simulink model "signal_proc"  (R2017a)
settings: Solver=VariableStepAuto  StartTime=0.0  StopTime=50  RelTol=1e-3  EnableMultiTasking=on
values from neighbouring files (symbols this model uses):
  Ts = 1/ Fs    (= 0.008)    [example_1.m]    (also in my_filter.m = 1/Fs)
libraries: dspsrcs4 x1
settings Model: Creator=haroldfmurcia  LastModifiedBy=root
settings OptimizationCC: LifeSpan=inf
settings DebuggingCC: SFUnexpectedBacktrackingDiag=warning  SFNoUnconditionalDefaultTransitionDiag=warning  SFExecutionAtInitializationDiag=none
settings GRTTargetCC: TargetLangStandard=C89/C90 (ANSI)  GeneratePreprocessorConditionals=Disable all
settings ConfigComp: CovMetricSettings=dw  CovHtmlReporting=on  CovSaveCumulativeToWorkspaceVar=on  CovSaveSingleToWorkspaceVar=on  CovExternalEMLEnable=off

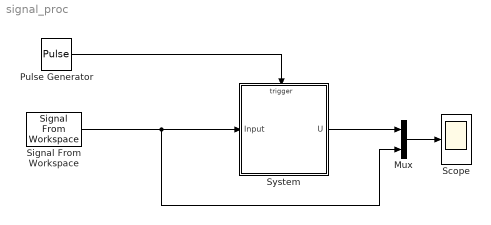
== system signal_proc ==
  Mux : Mux  Inputs=2
  Pulse Generator : DiscretePulseGenerator  PulseType=Time based  Period=Ts  PulseWidth=10
  Scope : Scope
  Signal From Workspace : dspsrcs4/Signal From Workspace  X=signal  Ts=Ts  nsamps=1  OutputAfterFinalValue=Setting to zero  ignoreOrWarnInputAndFrameLengths=off  OutputFrames=off
  System : Subsystem
  wires:
  Pulse Generator/1 -> System/Trigger
  Mux/1 -> Scope/1
  System/1(U) -> Mux/1
  Signal From Workspace/1 -> System/1(Input), Mux/2

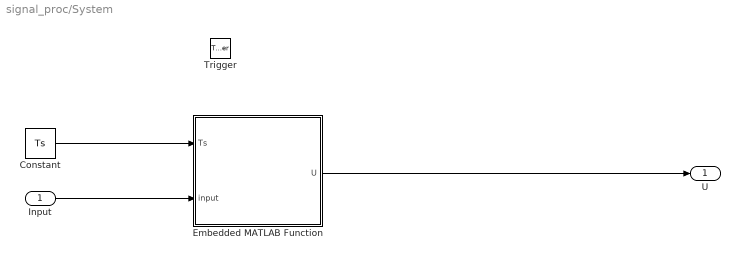
== system signal_proc/System ==
  Input : Inport
  Trigger : TriggerPort  VariantControl=Variant
  Constant : Constant  Value=Ts
  Embedded MATLAB Function : MATLAB Function  TreatAsAtomicUnit=on
  U : Outport
  wires:
  Embedded MATLAB Function/1(U) -> U/1
  Input/1 -> Embedded MATLAB Function/2(input)
  Constant/1 -> Embedded MATLAB Function/1(Ts)

== matlab function signal_proc/System/Embedded MATLAB Function ==
  data: Ts input; input input; U output
function U = fcn(Ts,input)
% Constants
B= [0.0815         0   -0.1630         0    0.0815];
A= [1.0000   -2.9862    3.3702   -1.7553    0.3722];

% Memory variables
persistent X_1 X_2 X_3 X_4  Y_1  Y_2 Y_3 Y_4 W samples;
if isempty(X_1) X_1=0;   end
if isempty(X_2) X_2=0;   end
if isempty(X_3) X_3=0;   end
if isempty(X_4) X_4=0;   end
if isempty(Y_1) Y_1=0;   end
if isempty(Y_2) Y_2=0;   end
if isempty(Y_3) Y_3=0;   end
if isempty(Y_4) Y_4=0;   end
if isempty(samples) samples=0;   end
if isempty(W) W=zeros(1,375);   end

% Variables
X=input;
X_vector = [X X_1 X_2 X_3 X_4];
Y_vector = [Y_1 Y_2 Y_3 Y_4];

% Main
samples = samples +1;
%Y = B(1)*X + B(2)*X_1 + B(3)*X_2 - A(2)*Y_1 - A(3)*Y_2;
Y = X_vector*B' - Y_vector*A(2:end)';

% Memory update
X_4=X_3;
X_3=X_2;
X_2=X_1;
X_1=X;
Y_4=Y_3;
Y_3=Y_2;
Y_2=Y_1;
Y_1=Y;


U=Y;
